simulink model "math_3_test"  (Simulink 7.2)
settings: Solver=VariableStepDiscrete  StartTime=0.0  StopTime=10.0  RelTol=1e-3
settings Model: Creator=arnaud  LastModifiedBy=arnaud
settings DataIOCC: SaveFormat=Structure

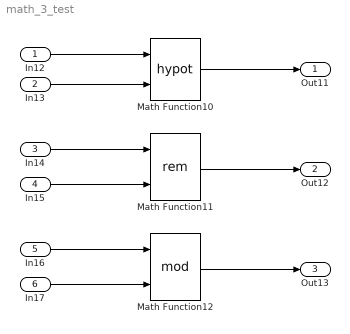
== system math_3_test ==
  In12 : Inport  OutDataType=sfix(16)  OutScaling=2^0
  In13 : Inport  Port=2  OutDataType=sfix(16)  OutScaling=2^0
  In14 : Inport  Port=3  OutDataType=sfix(16)  OutScaling=2^0
  In15 : Inport  Port=4  OutDataType=sfix(16)  OutScaling=2^0
  In16 : Inport  Port=5  OutDataType=sfix(16)  OutScaling=2^0
  In17 : Inport  Port=6  OutDataType=sfix(16)  OutScaling=2^0
  Math Function10 : Math  Operator=hypot  OutDataType=sfix(16)  OutScaling=2^0  SaturateOnIntegerOverflow=on
  Math Function11 : Math  Operator=rem  OutDataType=sfix(16)  OutScaling=2^0  SaturateOnIntegerOverflow=on
  Math Function12 : Math  Operator=mod  OutDataType=sfix(16)  OutScaling=2^0  SaturateOnIntegerOverflow=on
  Out11 : Outport  OutDataType=sfix(16)  OutScaling=2^0
  Out12 : Outport  Port=2  OutDataType=sfix(16)  OutScaling=2^0
  Out13 : Outport  Port=3  OutDataType=sfix(16)  OutScaling=2^0
  wires:
  In12/1 -> Math Function10/1
  In13/1 -> Math Function10/2
  Math Function10/1 -> Out11/1
  In14/1 -> Math Function11/1
  In15/1 -> Math Function11/2
  Math Function11/1 -> Out12/1
  In16/1 -> Math Function12/1
  In17/1 -> Math Function12/2
  Math Function12/1 -> Out13/1
